simulink model "slGTC_3gdl"  (Simulink 9.0)
settings: Solver=ode45  StartTime=0.0  StopTime=1  MaxStep=1e-3  RelTol=1e-8  EnableMultiTasking=on
settings Model: Creator=Manuel G. Ortega  LastModifiedBy=Raúl  ExtModeTrigMode=oneshot  ExtModeArmWhenConnect=off
settings DataIOCC: SignalLoggingSaveFormat=ModelDataLogs
settings OptimizationCC: BooleanDataType=off  ExpressionDepthLimit=2147483647  InitFltsAndDblsToZero=on
settings DebuggingCC: SaveWithParameterizedLinksMsg=none  SignalResolutionControl=TryResolveAllWithWarning  MultiTaskDSMMsg=warning  MultiTaskCondExecSysMsg=none  FcnCallInpInsideContextMsg=warning  StateNameClashWarn=warning  StrictBusMsg=None
settings HardwareCC: TargetUnknown=on
settings GRTTargetCC: TargetFcnLib=ansi_tfl_tmw.mat  GeneratePreprocessorConditionals=Disable all  CombineOutputUpdateFcns=off  GRTInterface=on
settings ConfigComp: CovSFcnEnable=off

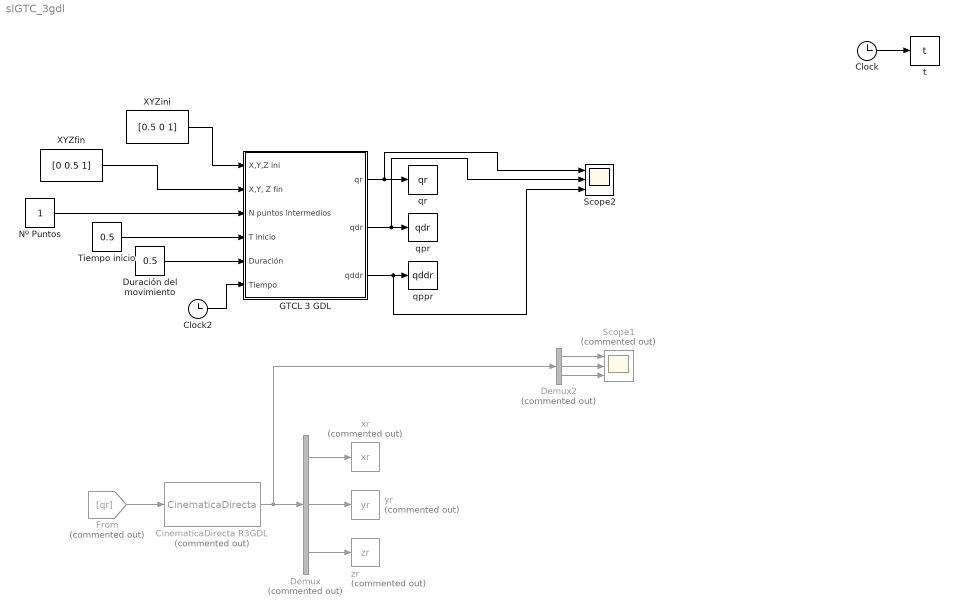
== system slGTC_3gdl ==
  CinematicaDirecta R3GDL : MATLABFcn  Commented=on  MATLABFcn=CinematicaDirecta
  Clock : Clock
  Clock2 : Clock
  Demux : Demux  Commented=on  Outputs=3
  Demux2 : Demux  Commented=on  Outputs=3
  Duración del movimiento : Constant  Value=0.5
  From : From  Commented=on  GotoTag=qr
      settings: CloseFcn=tagdialog Close
  GTCL 3 GDL : Subsystem
  Nº Puntos : Constant
  Scope1 : Scope  Commented=on  NumInputPorts=3
  Scope2 : Scope  NumInputPorts=3
  Tiempo inicio : Constant  Value=0.5
  XYZfin : Constant  Value=[0 0.5 1]
  XYZini : Constant  Value=[0.5 0 1]
  qppr : ToWorkspace  VariableName=qddr  SampleTime=-1
  qpr : ToWorkspace  VariableName=qdr  SampleTime=-1
  qr : ToWorkspace  VariableName=qr  SampleTime=-1
  t : ToWorkspace  VariableName=t  SampleTime=-1
  xr : ToWorkspace  Commented=on  VariableName=xr  SampleTime=-1
  yr : ToWorkspace  Commented=on  VariableName=yr  SampleTime=-1
  zr : ToWorkspace  Commented=on  VariableName=zr  SampleTime=-1
  wires:
  Clock/1 -> t/1
  Duración del movimiento/1 -> GTCL 3 GDL/5(Duración)
  Tiempo inicio/1 -> GTCL 3 GDL/4(T inicio)
  Nº Puntos/1 -> GTCL 3 GDL/3(N puntos intermedios)
  XYZfin/1 -> GTCL 3 GDL/2("X,Y, Z fin")
  XYZini/1 -> GTCL 3 GDL/1(X,Y,Z ini)
  From/1 -> CinematicaDirecta R3GDL/1
  CinematicaDirecta R3GDL/1 -> Demux2/1, Demux/1
  Demux/1 -> xr/1
  Demux/2 -> yr/1
  Demux/3 -> zr/1
  Demux2/3 -> Scope1/3
  Demux2/2 -> Scope1/2
  Demux2/1 -> Scope1/1
  GTCL 3 GDL/2(qdr) -> Scope2/2, qpr/1
  GTCL 3 GDL/1(qr) -> Scope2/1, qr/1
  GTCL 3 GDL/3(qddr) -> Scope2/3, qppr/1
  Clock2/1 -> GTCL 3 GDL/6(Tiempo)

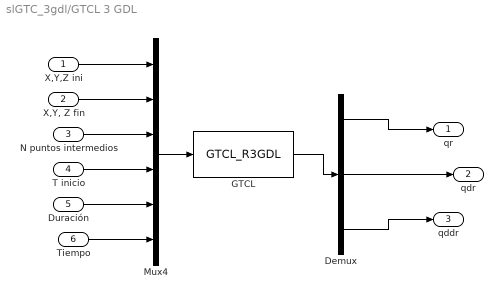
== system slGTC_3gdl/GTCL 3 GDL ==
  X,Y,Z ini : Inport
  "X,Y, Z fin" : Inport  Port=2
  N puntos intermedios : Inport  Port=3
  T inicio : Inport  Port=4
  Duración : Inport  Port=5
  Tiempo : Inport  Port=6
  Demux : Demux  Outputs=3
  GTCL : MATLABFcn  MATLABFcn=GTCL_R3GDL  OutputDimensions=3
  Mux4 : Mux  Inputs=6
  qr : Outport
  qdr : Outport  Port=2
  qddr : Outport  Port=3
  wires:
  Mux4/1 -> GTCL/1
  X,Y,Z ini/1 -> Mux4/1
  "X,Y, Z fin"/1 -> Mux4/2
  N puntos intermedios/1 -> Mux4/3
  T inicio/1 -> Mux4/4
  Duración/1 -> Mux4/5
  Tiempo/1 -> Mux4/6
  GTCL/1 -> Demux/1
  Demux/2 -> qdr/1
  Demux/1 -> qr/1
  Demux/3 -> qddr/1
